simulink model "Hybrid2_modified"  (R2025a)
settings: Solver=FixedStepAuto  StartTime=0.0  StopTime=1.0  FixedStep=Ts  RelTol=1e-3
undefined symbols (not defined in the file or in its folder): closedLoop, controller, D1, D11, Delta, DiscIntNeverNeededParam, find_system, grid, level, protection, sensor, solarPanel, solarPlant, Ts
libraries: powerlib_extras x38, nesl_utility x29, spsSampleandHoldLib x24, spsThyristorLib x24, spsSeriesRLCBranchLib x23, simulink x22, fl_lib x18, ee_lib x12, spsEdgeDetectorLib x12, spsParallelRLCBranchLib x10, spsThreePhaseVIMeasurementLib x9, simulink_extras x8
(part 1 of 8)
settings Model: Creator=ELMAN  LastModifiedBy=FX
settings OptimizationCC: SimCompilerOptimization=on

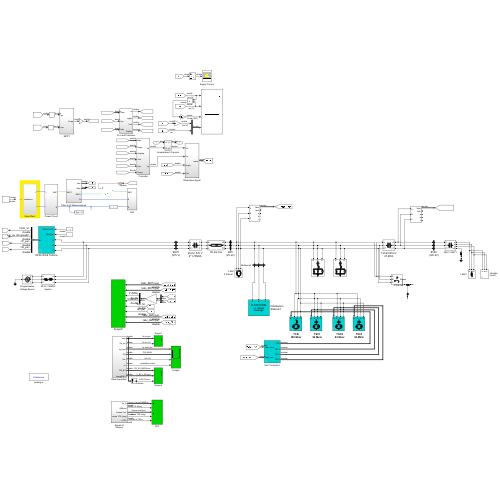
[thumbnail: Simulink's stored preview of the top-level diagram]
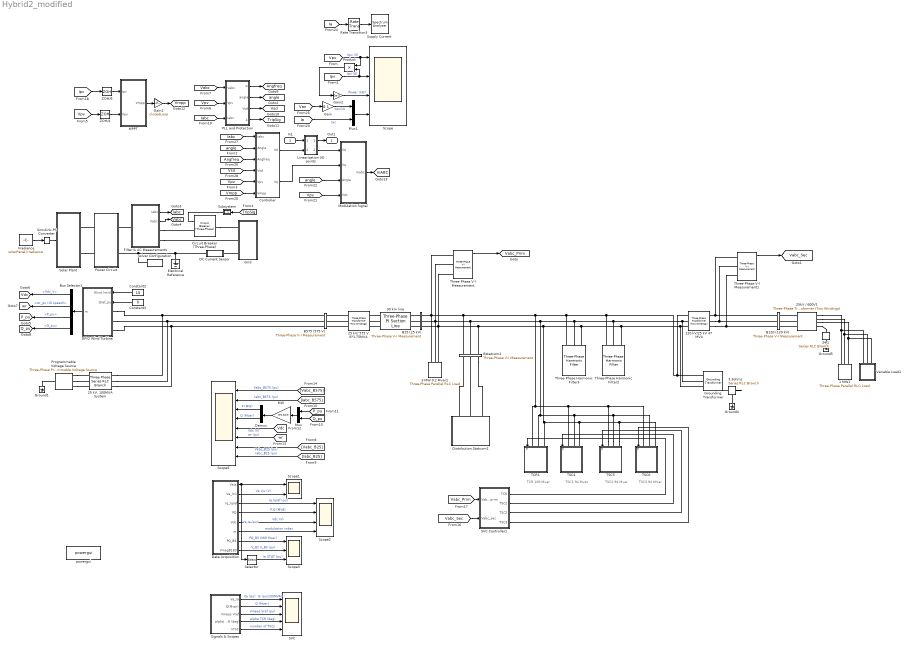
== system Hybrid2_modified ==
  note: TCR
      | 109 Mvar
  note: TSC1
      | 94 Mvar
  note: TSC2
      | 94 Mvar
  note: TSC3
      | 94 MVar
  In1 : Inport
  1 MW1 : spsThreePhaseParallelRLCLoadLib/Three-Phase Parallel RLC Load  LConnTagsString=A|B|C  Configuration=Y (floating)  NominalVoltage=600  Vabc=[1e3 1e3 1e3]  Vabcp=[1e3 1e3 1e3]  NominalFrequency=60  UnbalancedPower=off  ActivePower=1e6  InductivePower=0  CapacitivePower=0  Pabc=[10e3 9e3 11e3]  QLabc=[100 90 110]  QCabc=[100 90 110]  Pabcp=[10e3 9e3 11e3]  QLabcp=[100 90 110]  QCabcp=[100 90 110]  Measurements=None  LoadType=constant Z
  120 kV/25 kV 47 MVA : spsThreePhaseTransformerTwoWindingsLib/Three-Phase Transformer (Two Windings)  Winding1Connection=Yg  Winding2Connection=Delta (D1)  CoreType=Three single-phase transformers  SetSaturation=off  Hysteresis=off  DataFile='basic_model'  SetInitialFlux=off  Measurements=None  UNITS=pu  NominalPower=[47e6 60 ]  Winding1="[ 120e3  0.08/30   0.08 ]"  Winding2="[ 25e3  0.08/30  0.08]"  Rm=500  Lm=500  L0=0.5  Saturation="[ 0,0  ;  0.005,1.2  ;  1.0,1.4 ]"  InitialFluxes=[ 0.8 , -0.8 , 0.7 ]  BreakLoop=off  DiscreteSolver=Trapezoidal iterative  DataType=off  TransfoNumber=0
  "25 kV, 100MVA System" : spsThreePhaseSeriesRLCBranchLib/Three-Phase Series RLC Branch  LConnTagsString=A|B|C  RConnTagsString=A|B|C  BranchType=RL  Resistance=25e3^2/100e6/10  Inductance=25e3^2/100e6/(2*pi*60)  Capacitance=1.0  Measurements=None
  25 kV/ 575 V 6*1.75MVA : spsThreePhaseTransformerTwoWindingsLib/Three-Phase Transformer (Two Windings)  Winding1Connection=Delta (D11)  Winding2Connection=Yg  CoreType=Three single-phase transformers  SetSaturation=off  Hysteresis=off  DataFile='hysteresis'  SetInitialFlux=off  Measurements=None  UNITS=pu  NominalPower="[1.75e6*6  60]"  Winding1=[25e3 , 0.025/30 , 0.025]  Winding2=[ 575, 0.025/30 , 0.025]  Rm=500  Lm=inf  L0=0.5  Saturation=[ 0,0 ; 0.0024,1.2 ; 1.0,1.52 ]  InitialFluxes=[ 0.8 , -0.8 , 0.7 ]  BreakLoop=off  DiscreteSolver=Trapezoidal iterative  DataType=off  TransfoNumber=0
  25kV / 600V1 : spsThreePhaseTransformerTwoWindingsLib/Three-Phase Transformer (Two Windings)  Winding1Connection=Delta (D11)  Winding2Connection=Yn  CoreType=Three single-phase transformers  SetSaturation=off  Hysteresis=off  DataFile='basic_model'  SetInitialFlux=off  Measurements=None  UNITS=pu  NominalPower=[6e6 60]  Winding1=[25e3 , 0.05/30/2 , 0.05]  Winding2=[600 , 0.05/30/2 , 0]  Rm=500  Lm=500  L0=0.5  Saturation="[ 0,0  ;  0.005,1.2  ;  1.0,1.4 ]"  InitialFluxes=[ 0.8 , -0.8 , 0.7 ]  BreakLoop=off  DiscreteSolver=Trapezoidal iterative  DataType=off  TransfoNumber=1
  3 MW 0.2 Mvar1 : spsThreePhaseParallelRLCLoadLib/Three-Phase Parallel RLC Load  LConnTagsString=A|B|C  Configuration=Y (grounded)  NominalVoltage=25e3  Vabc=[1e3 1e3 1e3]  Vabcp=[1e3 1e3 1e3]  NominalFrequency=60  UnbalancedPower=off  ActivePower=3e6  InductivePower=0  CapacitivePower=0.2e6  Pabc=[10e3 9e3 11e3]  QLabc=[100 90 110]  QCabc=[100 90 110]  Pabcp=[10e3 9e3 11e3]  QLabcp=[100 90 110]  QCabcp=[100 90 110]  Measurements=None  LoadType=constant Z
  "3.3ohms " : spsSeriesRLCBranchLib/Series RLC Branch  LConnTagsString=__new0  RConnTagsString=__new0  BranchType=R  Resistance=3.3  Inductance=[]  SetiL0=off  InitialCurrent=0  Capacitance=[]  Setx0=off  InitialVoltage=0  Measurements=None
  30 km line : spsThreePhasePISectionLineLib/Three-Phase PI Section Line  LConnTagsString=a|b|c  RConnTagsString=A|B|C  Length=30  Frequency=60  Resistances=[0.1153 0.413]  Inductances=[1.05e-3 3.32e-3]  Capacitances=[11.33e-009 5.01e-009]
  34.1 : spsSeriesRLCBranchLib/Series RLC Branch  LConnTagsString=__new0  RConnTagsString=__new0  BranchType=R  Resistance=34.7  Inductance=1.0  SetiL0=off  InitialCurrent=0  Capacitance=1.0  Setx0=off  InitialVoltage=0  Measurements=None
  B120 (120 kV) : spsThreePhaseVIMeasurementLib/Three-Phase V-I Measurement  VoltageMeasurement=no  SetLabelV=off  LabelV=Vabc_B120  Vpu=off  VpuLL=off  CurrentMeasurement=no  SetLabelI=on  LabelI=Iabc_B120  Ipu=off  Pbase=100e6  Vbase=120e3  OutputType=Complex  PhasorSimulation=off  PSBequivalent=0
  B25 (25 kV) : spsThreePhaseVIMeasurementLib/Three-Phase V-I Measurement  VoltageMeasurement=phase-to-ground  SetLabelV=on  LabelV=Vabc_B25  Vpu=on  VpuLL=off  CurrentMeasurement=yes  SetLabelI=on  LabelI=Iabc_B25  Ipu=on  Pbase=10e6  Vbase=25e3  OutputType=Complex  PhasorSimulation=off  PSBequivalent=0
  B575 (575 V) : spsThreePhaseVIMeasurementLib/Three-Phase V-I Measurement  VoltageMeasurement=phase-to-ground  SetLabelV=on  LabelV=Vabc_B575  Vpu=on  VpuLL=off  CurrentMeasurement=yes  SetLabelI=on  LabelI=Iabc_B575  Ipu=on  Pbase=6*1.5e6/0.9  Vbase=575  OutputType=Complex  PhasorSimulation=off  PSBequivalent=0
  Bstatcom2 : spsThreePhaseVIMeasurementLib/Three-Phase V-I Measurement  VoltageMeasurement=phase-to-ground  SetLabelV=on  LabelV=Vabc_Bstatcom  Vpu=on  VpuLL=off  CurrentMeasurement=yes  SetLabelI=on  LabelI=Iabc_Bstatcom  Ipu=on  Pbase=3e6  Vbase=25e3  OutputType=Magnitude  PhasorSimulation=off  PSBequivalent=0
  Bus Selector1 : BusSelector  OutputSignals=Vdc_V,wr_pu (IG speed),PQ_pu.P_pu,PQ_pu.Q_pu
  Circuit Breaker (Three-Phase) : ee_lib/Switches & Breakers/Circuit Breaker (Three-Phase)  R_closed=0.0001 Ohm  G_open=1e-6 1/Ohm  threshold=0.5 V  breaker_behavior=ee.enum.switches.breakerBehavior.zeroCrossingEnable
      settings: InternalSimscapePortConfiguration="{\"Bottom\":[],\"Left\":[{\"id\":\"vT\",\"label\":\"vT\",\"type\":\"input\"},{\"id\":\"N1\",\"label\":\"~1\",\"type\":\"foundation.electrical.three_phase\"}],\"Right\":[{\"id\":\"N2\",\"label\":\"~2\",\"type\":\"foundation.electrical.three_phase\"}],\"Top\":[]}"
  Constant2 : Constant  Value=15
  Constant3 : Constant  Value=0
  Controller : Subsystem
  DC Current Sensor : Subsystem
      mask Display: disp('i')
  DFIG Wind Turbine : Subsystem  LoadFcn=%find_system(gcs,'FollowLinks', 'on', 'LookUnderMasks', 'all');  mask(DFIG Wind Turbine){Nb_wt=6, ShowParameters=Generator data for 1 wind turbine, nom=[1.5e6/.9 575 1975 60], sta=[ 0.023 0.18], rot=[ 0.016 0.16], Lm=2.9, mec=[0.685 0.01 3], init=[ -0.2,0   0,0,0   0,0,0 ], Imax_grid_conv=0.8, RL_grid=[ 0.3 0.003], Vdc_nom=1150, C_DClink1=10000e-6, C_var_filter1=120e3, Pmec1=1.5e6, wind_speed_CpMax=11, wind0=11, DisplayTurbChar=off, H_WT=4.32, Ksh=1.11, D_mutual=1.5, w_wt0=1.2, torque0=0.83, Kdc=[8   400], Kgrid_side_cur_reg=[0.83 5], Kspeed=[3 0.6], Krotor_side_cur_reg=[0.6 8], Ki_QV=[0.05 20], Kp_pitch=[150], Kcompensation=[3 30], PWM_freq_grid=2700, PWM_freq_rotor=1620, pitch_max=27, pitch_rate=10}
      mask prompts: Nb_wt "Number of wind turbines:"; ShowParameters "Display:"; nom "Nom. power, L-L volt. and freq. [Pn (VA), Vs_nom (Vrms), Vr_nom (Vrms), fn (Hz)]:"; sta "Stator [ Rs,Lls ] (p.u.):"; rot "Rotor [ Rr',Llr' ] (p.u.):"; Lm "Magnetizing inductance Lm (p.u.):"; mec "Inertia constant, friction factor, and pairs of poles [ H(s)  F(p.u.)  p ]:"; init "Initial conditions [s  th  ias  ibs  ics  phaseas phasebs phasecs]:"; Imax_grid_conv "Grid-side converter maximum current (pu of generator nominal current):"; RL_grid "Grid-side coupling inductor [ L, R] (p.u.):"; Vdc_nom "Nominal DC bus voltage (V):"; C_DClink1 "DC bus capacitor (F):"; C_var_filter1 "Line filter capacitor (Q=50) (var):"; Pmec1 "Nominal mechanical output power (W):"; wind_speed_CpMax "Wind speed at nominal speed and at Cp max (must be between 6 m/s and 30 m/s) (m/s):"; wind0 "Initial wind speed (m/s):"; DisplayTurbChar "Display wind turbine power characteristics:"; H_WT "Wind turbine inertia constant H (s):"; Ksh "Shaft spring constant refer to high-speed shaft (pu of nominal mechanical torque/rad):"; D_mutual "Shaft mutual damping (pu of nominal mechanical torque/pu dw):"; w_wt0 "Turbine initial speed (pu of nominal speed):"; torque0 "Initial output torque (pu of nominal mechanical torque):"; Kdc "DC bus voltage regulator gains [Kp Ki]:"; Kgrid_side_cur_reg "Grid-side converter current regulator gains [Kp Ki]:"; Kspeed "Speed regulator gains [Kp Ki]:"; Krotor_side_cur_reg "Rotor-side converter current regulator gains [Kp Ki]:"; Ki_QV "Q and V regulator gains [Ki_var Ki_volt]:"; Kp_pitch "Pitch controller gain [Kp]:"; Kcompensation "Pitch compensation gains [Kp Ki]:"; PWM_freq_grid "Frequency of the grid-side PWM carrier (Hz):"; PWM_freq_rotor "Frequency of the rotor-side PWM carrier (Hz):"; pitch_max "Maximum pitch angle (deg):"; pitch_rate "Maximum rate of change of pitch angle (deg/s):"
      mask help: This block implements a model of a variable speed pitch controlled wind turbine using a doubly-fed induction generator (DFIG).
      mask init:
      | %Generator data
      | Pnom=nom(1)*Nb_wt;
      | Vnom=nom(2);
      | Vnom_r=nom(3);
      | Fnom=nom(4);
      | Rs=sta(1);
      | Lls=sta(2);
      | Rr=rot(1);
      | Llr=rot(2);
      | H=mec(1);
      | F=mec(2);
      | p=mec(3);
      | 
      | % Converters data
      | L_RL=RL_grid(1);
      | R_RL=RL_grid(2);
      | Q_filter=50;
      | C_DClink=C_DClink1*Nb_wt;
      | C_var_filter=C_var_filter1*Nb_wt;
      | 
      | % Controller data
      | Freq_filter=1000*10;   %Hz
      | Zeta_filter=0.707;
      | Mod_index_max_grid=1.1;   %Maximum value of modulation index for grid-side converter
      | Mod_index_max_rotor=2;   %Maximum value of modulation index for rotor-side converter
      | Lim_grid_side_cur_reg=1.1; %Limit for grid-side PI current regulator (pu)
      | Lim_rotor_side_cur_reg=0.1; %Limit for rotor-side PI current regulator (pu)
      | Min_var_reg=0.9; %Minimum output value for integral var regulator (pu)
      | Max_var_reg=1.1; %Maximum output value for integral var regulator (pu)
      | Max_speed_reg=1; %Maximum output value for PI speed regulator (pu)
      | Kp_dc=Kdc(1);
      | Ki_dc=Kdc(2);
      | Kp_grid_side_cur_reg=Kgrid_side_cur_reg(1);
      | Ki_grid_side_cur_reg=Kgrid_side_cur_reg(2);
      | Kp_speed=Kspeed(1);
      | Ki_speed=Kspeed(2);
      | Kp_compensation=Kcompensation(1);
      | Ki_compensation=Kcompensation(2);
      | Kp_rotor_side_cur_reg=Krotor_side_cur_reg(1);
      | Ki_rotor_side_cur_reg=Krotor_side_cur_reg(2);
      | Ki_var=Ki_QV(1);
      | Ki_volt=Ki_QV(2);
      | Iq_ref_limit_time_constant=0.3; %(s)
      | T_speed=5;      %s
      | Min_mag_flux=0.5;   %(pu)
      | Max_Idr_ref=0.9;    %(pu)
      | Speed_max=1.2;  %(pu)
      | Speed_min=0.7;  %(pu)
      | Pitch_time_constant=0.01;    %(s)
      | 
      | 
      | % Turbine data
      | Pmec=Pmec1*Nb_wt;
      | c1 = 0.6450;
      | c2 = 116;
      | c3 = .4;
      | c4 = 5;
      | c5 = 21;
      | c6 = .00912;  % Set Pmin in stall condition (does not vary with wind_speed_Pmax)
      | c7 = .08;
      | c8 = .035;
      | theta=0;
      | CpMax=.5;
      | lambda_CpMax=9.9495;
      | 
      | c1_c8=[c1 c2 c3 c4 c5 c6 c7 c8];
      |   
      | 
      | %   Cp = c1*(c6*lambda + (-c4 - c3*(2.5 + theta) + c2*(1/(lambda + ...
      | %   c7*(2.5 + theta)) - c8/(1 + (2.5 + theta)^3)))/exp(c5*(1/(lambda + ...
      | %   c7*(2.5 + theta)) - c8/(1 + (2.5 + theta)^3))))
      | 
      | 
      |         %%%%%%%%%%%%%%%%%%%%%%%%%%%%%%%%%%%%%%%%%%%%%%%%%%%%%%%%%%%%%%%%%%%%%%%%%%%
      |         % Operation at Cp max
      |         %%%%%%%%%%%%%%%%%%%%%%%%%%%%%%%%%%%%%%%%%%%%%%%%%%%%%%%%%%%%%%%%%%%%%%%%%%%
      |         
      |         rated_omegar=1.2;
      |         omegar = rated_omegar;
      |         
      |         % Enforce boundaries on wind speed
      |         % A warning could be displayed
      |         if wind_speed_CpMax < 6
      |             wind_speed_CpMax=6;
      |             disp('Warning: Wind speed at nominal speed and at Cp max has been set to 6 m/s')
      |         end
      |         if wind_speed_CpMax > 30
      |             wind_speed_CpMax=30;
      |             disp('Warning: Wind speed at nominal speed and at Cp max has been set to 30 m/s')
      |         end
      | 
      |         K1=lambda_CpMax/omegar*wind_speed_CpMax;
      |         
      |         % Calculation of K2 needed to get P equal to the requested value at
      |         % Cp max for the requested wind speed
      |         
      |         Prated=Pmec1*Nb_wt;
      |         P_rated_omegar_theta_zero=0.75;
      |         
      |         K2 = P_rated_omegar_theta_zero*Prated/(wind_speed_CpMax^3*CpMax);
      |         
      |         K1_K2=[K1 K2];
      |         
      |         %%%%%%%%%%%%%%%%%%%%%%%%%%%%%%%%%%%%%%%%%%%%%%%%%%%%%%%%%%%%%%%%%%%%%%%%%%%
      |         % End of calculation for operation at Cp max
      |         %%%%%%%%%%%%%%%%%%%%%%%%%%%%%%%%%%%%%%%%%%%%%%%%%%%%%%%%%%%%%%%%%%%%%%%%%%%
      |         
      | 
      | %%%%%%%%%%%%%%%%%%%%%%%%%%%%%%%%%%%%%%%%%%%%%%%%%%%%%%%%%%%%%%%%%%%%%%%%%%%
      | % Plot turbine characteristics
      | %%%%%%%%%%%%%%%%%%%%%%%%%%%%%%%%%%%%%%%%%%%%%%%%%%%%%%%%%%%%%%%%%%%%%%%%%%% 
      | 
      | DisplayTurbChar=get_param(gcb,'DisplayTurbChar');
      | if strcmp(DisplayTurbChar,'on')
      |     vect_theta = 0:2:30;
      |     
      |     vect_lambda = 1:0.2:30;
      |     
      |     clear Cp;
      |     
      |     for i=1:length(vect_theta)
      |      for j=1:length(vect_lambda)
      |                 Cp(i,j) = c1*(c6*vect_lambda(j) + (-c4 - c3*(2.5 + vect_theta(i)) + c2*(1/(vect_lambda(j) + ...
      |                 c7*(2.5 + vect_theta(i))) - c8/(1 + (2.5 + vect_theta(i))^3)))/exp(c5*(1/(vect_lambda(j) + ...
      |                 c7*(2.5 + vect_theta(i))) - c8/(1 + (2.5 + vect_theta(i))^3))));
      |      end
      |     end
      | 
      |     figure(1);
      |     clf;
      |     hold on;
      | 
      |     plot(vect_lambda, Cp);
      |     axis([0, 25, 0, .6]);
      |     title('Wind Turbine Cp Characteristic (pitch angle increases by step of 2 deg.)');
      |     ylabel('Cp');
      |     set(gca,'ytick',[0 .1 .2 .3 .4 .5 .6]);
      |     xlabel('Lambda');
      |     grid on;
      |     text(10.1,0.51,'Pitch angle 0 degree');
      | 
      |     hold off
      |     
      |     % Plot of the wind turbine mechanical power output (pu) lambda and Cp
      |     % characteristics against wind speed (m/s) for a range of theta.
      |     
      |     wind_speed_range = [1,.2,30];
      |     vect_wind_speed = 1:0.2:30;
      |     
      |     clear lambda;
      |     clear Cp;
      |     clear P;
      | 
      |     for i=1:length(vect_theta)
      |         for j=1:length(vect_wind_speed)
      |             lambda(i,j) = K1*omegar/vect_wind_speed(j);
      |             Cp(i,j) = c1*(c6*lambda(i,j) + (-c4 - c3*(2.5 + vect_theta(i)) + c2*(1/(lambda(i,j) + ...
      |             c7*(2.5 + vect_theta(i))) - c8/(1 + (2.5 + vect_theta(i))^3)))/exp(c5*(1/(lambda(i,j) + ...
      |             c7*(2.5 + vect_theta(i))) - c8/(1 + (2.5 + vect_theta(i))^3))));
      |             P(i,j) = K2/Prated*vect_wind_speed(j)^3*Cp(i,j);
      |         end
      |     end
      |     
      |     
      |     figure(2);
      |     clf;
      |     hold on
      |     
      |     subplot(3,1,1);
      |     plot(vect_wind_speed, P);
      |     axis([0, 35, 0, 1.5]);
      |     title('Wind Turbine Characteristics (w = 1.2 pu, pitch angle increases by step of 2 deg.)');
      |     ylabel('P (pu)');
      |     set(gca,'ytick',0:.5:4);
      |     grid on;
      |     
      |     subplot(3,1,2);
      |     plot(vect_wind_speed, lambda);
      |     axis([0, 35, 0, 20]);
      |     ylabel('Lambda');
      |     grid on;
      |     
      |     subplot(3,1,3)
      |     plot(vect_wind_speed, Cp);
      |     axis([0, 35, 0, .6]);
      |     xlabel('Wind Speed (m/s)');
      |     ylabel('Cp');
      |     set(gca,'ytick',[0 .1 .2 .3 .4 .5 .6]);
      |     grid on;
      | 
      |     hold off
      |     set_param(gcb,'DisplayTurbChar','off')
      |     
      | end
      mask TypeOptions ShowParameters: Generator data for 1 wind turbine | Converters data for 1 wind turbine | Turbine data for 1 wind turbine | Drive train data for 1 wind turbine | Control parameters for 1 wind turbine
      mask Callback ShowParameters:
      | BlockName=getfullname(gcb);
      | %
      | Param_Show=get_param(BlockName,'ShowParameters');
      | Param_DisplayTurbChar=get_param(BlockName,'DisplayTurbChar');
      | 
      | p_mask{3}='off';p_mask{4}='off';p_mask{5}='off';
      | p_mask{6}='off';p_mask{7}='off';p_mask{8}='off';p_mask{9}='off';
      | p_mask{10}='off';p_mask{11}='off';p_mask{12}='off';p_mask{13}='off';
      | p_mask{14}='off';p_mask{15}='off';p_mask{16}='off';p_mask{17}='off';
      | p_mask{18}='off';p_mask{19}='off';p_mask{20}='off';p_mask{21}='off';
      | p_mask{22}='off';p_mask{23}='off';p_mask{24}='off';p_mask{25}='off';
      | p_mask{26}='off';p_mask{27}='off';p_mask{28}='off';p_mask{29}='off';
      | p_mask{30}='off';p_mask{31}='off';p_mask{32}='off';p_mask{33}='off';
      | 
      | 
      | switch Param_Show
      | 	case 'Generator data for 1 wind turbine'
      | 		p_mask{3}='on';p_mask{4}='on';p_mask{5}='on'; p_mask{6}='on';
      |         p_mask{7}='on'; p_mask{8}='on';
      |     case 'Converters data for 1 wind turbine'
      | 		p_mask{9}='on';p_mask{10}='on';p_mask{11}='on';p_mask{12}='on';
      |         p_mask{13}='on';
      | 	case 'Turbine data for 1 wind turbine'
      |         p_mask{14}='on';p_mask{15}='on';p_mask{16}='on';p_mask{17}='on';
      |     case 'Drive train data for 1 wind turbine'
      |         p_mask{18}='on';p_mask{19}='on';p_mask{20}='on';p_mask{21}='on';
      |         p_mask{22}='on';
      |     case 'Control parameters for 1 wind turbine'
      |         p_mask{23}='on';p_mask{24}='on';p_mask{25}='on';
      |         p_mask{26}='on';p_mask{27}='on';p_mask{28}='on';p_mask{29}='on';
      |         p_mask{30}='on'; p_mask{31}='on';p_mask{32}='on'; p_mask{33}='on';
      | end
      | 
      | ParVisible={'on','on',p_mask{3},p_mask{4},p_mask{5},p_mask{6},p_mask{7},...
      |     p_mask{8},p_mask{9},p_mask{10},p_mask{11},p_mask{12},p_mask{13},...
      |     p_mask{14},p_mask{15},p_mask{16},p_mask{17},p_mask{18},p_mask{19},...
      |     p_mask{20},p_mask{21},p_mask{22},p_mask{23},p_mask{24},p_mask{25},...
      |     p_mask{26},p_mask{27},p_mask{28},p_mask{29},p_mask{30},p_mask{31},...
      |     p_mask{32},p_mask{33}};
      | %
      | set_param(BlockName,'MaskVisibilities',ParVisible);
      | set_param(BlockName,'DisplayTurbChar',Param_DisplayTurbChar);
  Data Acquisition : Subsystem
  Demux : Demux  Outputs=2
  Distribution Statcom1 : Subsystem
      mask Display: disp('D-STATCOM\n+/- 3Mvar\nAverage')
  Electrical Reference : fl_lib/Electrical/Electrical Elements/Electrical Reference
  Filter & AC Measurements : Subsystem
  Gain : Gain  Gain=0.1
  Gain1 : Gain  Gain=closedLoop
  Gain2 : Gain  Gain=1e-3
  Grid : Subsystem
  Ground1 : spsGroundLib/Ground  LConnTagsString=a
  Ground4 : spsGroundLib/Ground  LConnTagsString=a
  Ground5 : spsGroundLib/Ground  LConnTagsString=a
  "Grounding Transformer " : spsGroundingTransformerLib/Grounding Transformer   UNITS=pu  NominalPower="[100e6   60]"  NominalVoltage=25e3  ZeroSequenceImpedance_pu=[0.025 0.75]  MagnetizationBranch_pu=[500 500]  ZeroSequenceImpedance_SI=[0.052083 589.05]  MagnetizationBranch_SI=[1041.7 3.927e+005]  Measurements=None
  Irradiance : Constant  Value=solarPanel.irradiance
  Linearization I/O points : Subsystem
  MPPT : Subsystem
  MW : Gain  Gain=6*1.5/0.9  SaturateOnIntegerOverflow=on  OutDataTypeStr=Inherit: Same as input  ParamDataTypeStr=Inherit: Same as input
  Modulation Signal : Subsystem
  Mux : Mux  Inputs=2
  Mux1 : Mux  Inputs=2
  PLL and Protection : Subsystem
  Power Circuit : Subsystem
  Product : Product
  Programmable Voltage Source : spsThreePhaseProgrammableVoltageSourceLib/Three-Phase Programmable Voltage Source  PositiveSequence=[1.077*25e3 19 60]  VariationEntity=Amplitude  VariationType=Table of time-amplitude pairs  VariationTypeAlt=Step  VariationStep=0.5  VariationRate=10  VariationMagnitude=0.3  VariationFrequency=2  VariationTiming=[1 2]  VariationPhaseA=off  Amplitudes=[1 1.06 0.94 1.0]  TimeValues="[0 0.2  0.3   0.4 ]"  HarmonicGeneration=off  HarmonicA=[3 0.2 -25 0]  HarmonicB=[2 0.15 35 2]  Timing="[0.05  3]"  BusType=swing  Pref=0  Qref=0  Qmin=-inf  Qmax=inf
  Rate Transition3 : RateTransition  OutPortSampleTime=1/(5*solarPlant.switchFrequency)
  SVC : Scope  NumInputPorts=5
      settings: SampleTime=Ts  TimeSpan=0.5993512312472854  ActiveDisplayYMinimum=-4  ActiveDisplayYMaximum=4  DataLoggingVariableName=VIabc_Prim
  SVC Controller1 : Subsystem  mask(SVC Controller){OpMode=Voltage regulation, Vref=1.0, KpKi=[0 800], Xs=0.01, Bmin_max=[-1.04  3.23], Bref=0, Ts=Ts}
      mask prompts: OpMode "Operation mode"; Vref "Reference voltage (pu):"; KpKi "Regulator gains [ Kp  Ki ]:"; Xs "Droop (pu/100MVA):"; Bmin_max "Min. and max. primary susceptances [ Bind Bcap] (pu/100MVA):"; Bref "Susceptance Bref (pu/100MVA) (Var control mode):"; Ts "Sample time (s):"
      mask help:
      | This block implements a controller for a Static Var Compensator (SVC) consisting of one thyristor-controlled reactor bank (TCR) and three thyristor-switched capacitor banks (TSCs). Outputs TCR, TSC1, TSC2 and TSC3 are vectors of six pulses for the TCR and the three TSCs.
      | In Voltage control mode the primary voltage (Vabc_prim) is controlled at Vref within the maximum inductive and capacitive susceptance range and droop setting. In Var control mode the SVC susceptance  is  kept constant at Bref (Bref<0 for inductive mode).
      | Thyristor pulses are synchronized on secondary line-to-line voltages (Vabc_sec) of the coupling transformer, assuming a Wye/Delta (D1) connection.
      mask init:
      | Kp=KpKi(1);
      | Ki=KpKi(2);
      | Bmin=Bmin_max(1);
      | Bmax=Bmin_max(2);
      mask TypeOptions OpMode: Voltage regulation | Var control (Fixed susceptance Bref)
  Scope : Scope  NumInputPorts=4
      settings: TimeSpan=simulation.timeSim  ActiveDisplayYMinimum=-178.21524004215382  ActiveDisplayYMaximum=1603.9371603793847
  Scope1 : Scope  NumInputPorts=2
      settings: SampleTime=Ts  TimeSpan=0.5  ActiveDisplayYMinimum=-1.5  ActiveDisplayYMaximum=1.5  DataLoggingVariableName=Sig1
  Scope2 : Scope  NumInputPorts=4
      settings: SampleTime=Ts*32  TimeSpan=0.5  ActiveDisplayYMinimum=-2.0010436377768239  ActiveDisplayYMaximum=1.7915582294498202  DataLoggingVariableName=Sig2
  Scope3 : Scope  NumInputPorts=3
      settings: SampleTime=Ts  TimeSpan=0.5  ActiveDisplayYMinimum=-1  ActiveDisplayYMaximum=1  DataLoggingVariableName=Sig
  Scope5 : Scope  NumInputPorts=8
      settings: TimeSpan=0.2  ActiveDisplayYMinimum=-2  ActiveDisplayYMaximum=2  DataLoggingVariableName=ScopeData2  DataLoggingSaveFormat=Array
  Selector : Selector  InputPortWidth=2  IndexOptions=Index vector (dialog)  Indices=2  OutputSizes=1
  Signals & Scopes : Subsystem
  Simulink-PS Converter : nesl_utility/Simulink-PS Converter  PhysicalDomain=network_engine_domain  SubClassName=ps_input  LeftPortType=input  RightPortType=output  PseudoPeriodic=off  Frequencies=[]  NoiseDistribution=none  NoiseParameters=[]  Unit=1  AffineConversion=off  FilteringAndDerivatives=provide  SimscapeFilterOrder=1  InputFilterTimeConstant=0.001  UdotUserProvided=0
  Solar Plant : Subsystem
  Solver Configuration : nesl_utility/Solver Configuration  PhysicalDomain=network_engine_domain  SubClassName=solver  LeftPortType=input  RightPortType=generic  Tones=[]  Harmonics=[]  SimulateNoise=off  Profile=off  UseLocalSampling=off  EnableSwitchedLinearOptims=on  FrequencyDomain=off  UseCCode=off  RelTol=0.001  AbsTol=1e-06  MinStep=1e-09  ToWorkspace=off  RevertToSquareIcSolve=off  NumHomotopyIterations=100  PhasorMode=off  PhasorModeNumHarmonics=1  ConsistencySolver=NEWTON_FTOL  IndexReductionMethod=DerivativeReplacement  DoDC=off  ResidualTolerance=1e-9  ConsistencyTolSource=GLOBAL  ConsistencyAbsTol=0.001  ConsistencyRelTol=0.001  ConsistencyTolFactor=0.001  UseLocalSolver=off  LocalSolverChoice=NE_TRAPEZOIDAL_ADVANCER  ResolveIndetEquations=on  FunctionEvalNumThread=1  LocalSolverSampleTime=1e-7  DoFixedCost=off  MaxNonlinIter=10  MaxModeIter=2  ComputeImpulses=off  ImpulseIterations=2  LinearAlgebra=auto  LinearAlgebraNumThread=0  EquationFormulation=NE_TIME_EF  DelaysMemoryBudget=1024  AutomaticFiltering=on  FilteringTimeConstant=0.001  PartitionStorageMethod=AS_NEEDED  PartitionMemoryBudget=1024  PartitionMethod=FAST  MultibodyUseLocalSolver=off  MultibodyLocalSolverChoice=ODE1  MultibodyLocalSolverSampleTime=0.001
  Subsystem : Subsystem
  Supply Current : SpectrumAnalyzer  WindowPosition=[1059 553 620 438]  ScopeFrameLocation=window  SpectrumType=RMS  Method=Welch  SampleRate=100000  PlotAsTwoSidedSpectrum=off  FrequencyScale=Log  AxesScaling=Manual  RBWSource=Property  RBW=9  Span=50000  CenterFrequency=25000  StartFrequency=0  StopFrequency=50000  OverlapPercent=90  AveragingMethod=Running  SpectrumUnits=Vrms  YLimits=[-4.5063154233397524351,40.557285835884592018]  ColorLimits=[0.0061790664803535039207,16.888204283875005274]  AllowFFTLengthLessThanSamplesPerUpdate=on
      settings: OpenAtSimulationStart=off
  TCR1 : Subsystem  LoadFcn=find_system(gcs,'FollowLinks', 'on', 'LookUnderMasks', 'all');  mask(TCR branch){Ltcr=18.7e-3, Q=50, ParS=[500 250e-9], ParT=[1e-3  1*15]}
      mask prompts: Ltcr "TCR Inductance (H) :"; Q "Quality factor:"; ParS "Thyristor snubber: [ R (ohm)   C (F)  ]"; ParT "Thyristor data: [ Ron (ohm)   Vf (volt) ]"
      mask init:
      | Rtcr=(2*pi*60) * Ltcr / Q;
      | Rsnub=ParS(1);
      | Csnub=ParS(2);
      | Ron=ParT(1);
      | Vf=ParT(2);
      mask Display:
      | plot(0,0);plot(125,220)
      | plot([62 62 37 37 49 25 37],[15 39 39 58 76 76 58])
      | plot([62 87 87 99 87 75 87],[39 39 58 58 76 58 58])
      | plot([25 49],[58 58]);plot([37 25],[58 49])
      | plot([75 99],[76 76]);plot([87 99],[76 85])
      | plot([37 37 87 87],[76 95 95 76])
      | plot([62 62],[95 122]);plot([62 62],[164 186])
      | plot([62 72 78 79 78 72 62],[122 123 125 129 133 135 136])
      | plot([62 72 78 79 78 72 62],14+[122 123 125 129 133 135 136])
      | plot([62 72 78 79 78 72 62],28+[122 123 125 129 133 135 136])
  TSC4 : Subsystem  mask(TSC branch){Ccmt=308.4e-6, ParL=[1.13e-3 4.26e-3*2 191.7/2], ParS=[500 250e-9], ParT=[1e-3  1*15]}
      mask prompts: Ccmt "Capacitance (F) :"; ParL "[ Inductance (H)  Rseries (ohm)  Rparallel (ohm)  ]"; ParS "Thyristor snubber: [ R (ohm)   C (F)  ]"; ParT "Thyristor data: [ Ron (ohm)  Vf (volt) ]"
      mask init:
      | Lcmt=ParL(1);
      | Rseries=ParL(2);
      | Rparallel=ParL(3);
      | Rsnub=ParS(1);
      | Csnub=ParS(2);
      | Ron=ParT(1);
      | Vf=ParT(2);
      mask Display:
      | plot(0,0);plot(125,220)
      | plot([62 62 37 37 49 25 37],[15 39 39 58 76 76 58])
      | plot([62 87 87 99 87 75 87],[39 39 58 58 76 58 58])
      | plot([25 49],[58 58]);plot([37 25],[58 49])
      | plot([75 99],[76 76]);plot([87 99],[76 85])
      | plot([37 37 87 87],[76 95 95 76])
      | plot([62 62],[95 133]);plot([62 62],[164 183])
      | plot([62 69 73 78 81 82],13+[120 120 119 118 117 115])
      | plot([62 55 51 46 43 42],13+[120 120 119 118 117 115])
      | plot([42 82],[145 145])
      | plot([62 62],[145 164])
  TSC5 : Subsystem  mask(TSC branch){Ccmt=308.4e-6, ParL=[1.13e-3 4.26e-3*2 191.7/2], ParS=[500 250e-9], ParT=[1e-3 1*15]}
      mask prompts: Ccmt "Capacitance (F) :"; ParL "[ Inductance (H)  Rseries (ohm)  Rparallel (ohm)  ]"; ParS "Thyristor snubber: [ R (ohm)   C (F)  ]"; ParT "Thyristor data: [ Ron (ohm)  Vf (volt) ]"
      mask init:
      | Lcmt=ParL(1);
      | Rseries=ParL(2);
      | Rparallel=ParL(3);
      | Rsnub=ParS(1);
      | Csnub=ParS(2);
      | Ron=ParT(1);
      | Vf=ParT(2);
      mask Display:
      | plot(0,0);plot(125,220)
      | plot([62 62 37 37 49 25 37],[15 39 39 58 76 76 58])
      | plot([62 87 87 99 87 75 87],[39 39 58 58 76 58 58])
      | plot([25 49],[58 58]);plot([37 25],[58 49])
      | plot([75 99],[76 76]);plot([87 99],[76 85])
      | plot([37 37 87 87],[76 95 95 76])
      | plot([62 62],[95 133]);plot([62 62],[164 183])
      | plot([62 69 73 78 81 82],13+[120 120 119 118 117 115])
      | plot([62 55 51 46 43 42],13+[120 120 119 118 117 115])
      | plot([42 82],[145 145])
      | plot([62 62],[145 164])
  TSC6 : Subsystem  mask(TSC branch){Ccmt=308.4e-6, ParL=[1.13e-3 4.26e-3*2 191.7/2], ParS=[500 250e-9], ParT=[1e-3 1*15]}
      mask prompts: Ccmt "Capacitance (F) :"; ParL "[ Inductance (H)  Rseries (ohm)  Rparallel (ohm)  ]"; ParS "Thyristor snubber: [ R (ohm)   C (F)  ]"; ParT "Thyristor data: [ Ron (ohm)  Vf (volt) ]"
      mask init:
      | Lcmt=ParL(1);
      | Rseries=ParL(2);
      | Rparallel=ParL(3);
      | Rsnub=ParS(1);
      | Csnub=ParS(2);
      | Ron=ParT(1);
      | Vf=ParT(2);
      mask Display:
      | plot(0,0);plot(125,220)
      | plot([62 62 37 37 49 25 37],[15 39 39 58 76 76 58])
      | plot([62 87 87 99 87 75 87],[39 39 58 58 76 58 58])
      | plot([25 49],[58 58]);plot([37 25],[58 49])
      | plot([75 99],[76 76]);plot([87 99],[76 85])
      | plot([37 37 87 87],[76 95 95 76])
      | plot([62 62],[95 133]);plot([62 62],[164 183])
      | plot([62 69 73 78 81 82],13+[120 120 119 118 117 115])
      | plot([62 55 51 46 43 42],13+[120 120 119 118 117 115])
      | plot([42 82],[145 145])
      | plot([62 62],[145 164])
  Three-Phase Harmonic Filter2 : spsThreePhaseHarmonicFilterLib/Three-Phase Harmonic Filter  LConnTagsString=A|B|C  RConnTagsString=n  FilterType=Double-tuned  FilterConnection=Y (neutral)  ParNom=[315e3 60]  Qc=49e6  Fr=[5*60]  Frd=[11*60 13*60]  Q=16  Measurements=None
      settings: AttributesFormatString=\n
      settings: LibrarySourceBlock=|
      | sps_lib/Passives/Three-Phase
      | Harmonic Filter
  Three-Phase Harmonic Filter3 : spsThreePhaseHarmonicFilterLib/Three-Phase Harmonic Filter  LConnTagsString=A|B|C  RConnTagsString=n  FilterType=Double-tuned  FilterConnection=Y (neutral)  ParNom=[315e3 60]  Qc=49e6  Fr=[5*60]  Frd=[11*60 13*60]  Q=16  Measurements=None
      settings: AttributesFormatString=\n
      settings: LibrarySourceBlock=|
      | sps_lib/Passives/Three-Phase
      | Harmonic Filter
  Three-Phase V-I Measurement : spsThreePhaseVIMeasurementLib/Three-Phase V-I Measurement  VoltageMeasurement=phase-to-ground  SetLabelV=off  LabelV=Vabc  Vpu=off  VpuLL=off  CurrentMeasurement=yes  SetLabelI=off  LabelI=Iabc  Ipu=off  Pbase=100e6  Vbase=500e3  OutputType=Complex  PhasorSimulation=off  PSBequivalent=0
  Three-Phase V-I Measurement1 : spsThreePhaseVIMeasurementLib/Three-Phase V-I Measurement  VoltageMeasurement=phase-to-ground  SetLabelV=off  LabelV=Vabc  Vpu=off  VpuLL=off  CurrentMeasurement=yes  SetLabelI=off  LabelI=Iabc  Ipu=off  Pbase=100e6  Vbase=500e3  OutputType=Complex  PhasorSimulation=off  PSBequivalent=0
  Variable Load1 : Subsystem  mask(Variable Load (Constant Current)){Par_Nom=[3000 0.9], Par_Mod=[2000  5], Par_Time=[0.15 1]*100, Vbase=600, Ts=Ts}
      mask prompts: Par_Nom "Nominal load: [ Current (Arms)    Power factor (0 a 1) ]"; Par_Mod "Modulation: [ Amplitude (Arms)   Frequency (Hz) ]"; Par_Time "Modulation timing : [ Ton  Toff ]"; Vbase "Nominal voltage (Volts rms ph-ph)"; Ts "Sample time:"
      mask init:
      | NomAmp=Par_Nom(1)*sqrt(2);
      | NomPha=-acos(Par_Nom(2));
      | ModFreq=Par_Mod(2);
      | ModAmp=Par_Mod(1)*sqrt(2);
      | Ton=Par_Time(1);
      | Toff=Par_Time(2);
  ZOH/4 : ZeroOrderHold  SampleTime=solarPlant.timeMPPT
  ZOH/6 : ZeroOrderHold  SampleTime=solarPlant.timeMPPT
  powergui : spspowerguiLib/powergui  Priority=2  SimulationMode=Continuous  SampleTime=Ts  frequency=60  Iterations=50  frequencyindice=0  Pbase=100e6  ErrMax=1e-4  UnitsV=kV  UnitsW=MW  buscounter=0  FunctionMessages=off  echomessages=off  EnableUseOfTLC=off  CurrentSourceSwitches=off  DisableSnubberDevices=off  DisableRonSwitches=off  DisableVfSwitches=off  DisplayEquations=off  AutomaticDiscreteSolvers=off  SolverType=Tustin/Backward Euler (TBE)  Interpol=off  ExternalGateDelay=off  methode=off  Ts=0  x0status=blocks  SPID=off  SwTol=0  HookPort=off  NonlinearTolerance=1e-4  nMaxIteration=100  ContinueOnMaxIteration=off  RestoreLinks=warning  ResistiveCurrentMeasurement=off  Frange=[0:2:500]  Ylog=off  Xlog=on  ShowGrid=off  save=off  variable=ZData  structure=Sig1  ZoomFFT=on  StartTime=0.26  cycles=2  DisplayStyle=1  fundamental=60  FreqAxis=off  MaxFrequency=5000  frequencyindicesteady=1  RmsSteady=1  display=off
  Out1 : Outport  VectorParamsAs1DForOutWhenUnconnected=off
  tag scope: Angfreq=global, Iabc=global, P_pu=global, Q_pu=global, TripSig=global, Vabc=global, Vabc_Prim=global, Vabc_Sec=global, Vdc=global, Vmpp=global, Vsd=global, angle=global, mABC=global, wr=global
  wires:
  Selector/1 -> Scope3/3  "Ia STAT (pu)"
  Data Acquisition/8(VmagB1B3) -> Scope3/2  "V_B1 V_B3 (pu)"
  Data Acquisition/6(m) -> Scope2/4  "modulation index"
  Data Acquisition/4(PQ) -> Scope2/2  "P,Q (MVA)"
  Data Acquisition/1(VaIa) -> Scope1/1, Selector/1  "Va,Ia (pu)"
  Data Acquisition/3(Iq_Iqref) -> Scope2/1  "Iq,Iqref (pu)"
  Data Acquisition/2(Va_Inv) -> Scope1/2  "Va Inv (V)"
  Data Acquisition/5(Vdc) -> Scope2/3  "Vdc (V)"
  Data Acquisition/7(PQ_B3) -> Scope3/1  "PQ_B3 (MW Mvar)"
  Signals & Scopes/3("Vmeas Vref ") -> SVC/3  "Vmeas Vref (pu)"
  Signals & Scopes/4(alpha TCR (deg)) -> SVC/4  "alpha TCR (deg)"
  Signals & Scopes/5(nTSC) -> SVC/5  "number of TSCs"
  Signals & Scopes/2(Q(Mvar)) -> SVC/2  "Q (Mvar)"
  Signals & Scopes/1(Va_Ia) -> SVC/1  "Va (pu)  Ia (pu/100MVA)"
  DFIG Wind Turbine/1(m) -> Bus Selector1/1
  [Iabc_B575] -> Scope5/2  "Iabc_B575 (pu)"
  [P_pu] -> Mux/1
  Bus Selector1/4 -> [Q_pu]  "<Q_pu>"
  Bus Selector1/3 -> [P_pu]  "<P_pu>"
  Mux/1 -> MW/1
  [wr] -> Scope5/6  "wr (pu)"
  Demux/1 -> Scope5/3  "P (MW)"
  Bus Selector1/1 -> [Vdc]  "<Vdc_V>"
  [Iabc_B25] -> Scope5/8  "Iabc_B25 (pu)"
  Bus Selector1/2 -> [wr]  "<wr_pu (IG speed)>"
  [Q_pu] -> Mux/2
  [Vdc] -> Scope5/5  "Vdc (V)"
  Demux/2 -> Scope5/4  "Q (Mvar)"
  [Vabc_B575] -> Scope5/1  "Vabc_B575 (pu)"
  Constant2/1 -> DFIG Wind Turbine/1("Wind (m/s) ")
  [Vabc_B25] -> Scope5/7  "Vabc_B25 (pu)"
  Constant3/1 -> DFIG Wind Turbine/2(Qref_pu)
  MW/1 -> Demux/1
  SVC Controller1/4(TSC3) -> TSC6/1(P)
  SVC Controller1/3(TSC2) -> TSC5/1(P)
  SVC Controller1/1(TCR) -> TCR1/1(P)
  SVC Controller1/2(TSC1) -> TSC4/1(P)
  [Vabc_Sec] -> SVC Controller1/2(Vabc_sec)
  [Vabc_Prim] -> SVC Controller1/1(Vabc_prim)
  Three-Phase V-I Measurement/1 -> [Vabc_Prim]
  Three-Phase V-I Measurement1/1 -> [Vabc_Sec]
  [Vpv] -> Controller/5(Vpv)
  [Ipv] -> ZOH/6/1
  Modulation Signal/1(mabc) -> [mABC]
  [Vsd] -> Controller/4(Vsd)
  [Angfreq] -> Controller/3(Angfreq)
  Mux1/1 -> Scope/4
  Filter & AC Measurements/1(Iabc) -> [Iabc]
  [angle] -> Controller/2(Angle)
  [Vabc] -> PLL and Protection/1(Vabc)
  [Vpv] -> ZOH/4/1
  [Van] -> Gain/1
  PLL and Protection/4(TripSig) -> [TripSig]
  Linearization I/O points/2(y1) -> Modulation Signal/1(Vd)
  Gain1/1 -> [Vmpp]
  ZOH/4/1 -> MPPT/2(Vpv)
  Linearization I/O points/1(y2) -> Out1/1
  Irradiance/1 -> Simulink-PS Converter/1
  [angle] -> Modulation Signal/3(Angle)
  [Vpv] -> Product/1, Scope/1  "Vpv (V)"
  Gain2/1 -> Scope/3  "Power (kW)"
  Controller/2(Vq) -> Modulation Signal/2(Vq)
  [Vpv] -> PLL and Protection/2(Vpv)
  MPPT/1(Vmpp) -> Gain1/1
  PLL and Protection/1(w) -> [Angfreq]
  Filter & AC Measurements/2(Vabc) -> [Vabc]
  [TripSig] -> Subsystem/1(i)
  PLL and Protection/2(angle) -> [angle]
  [Iabc] -> Controller/1(Iabc)
  [Ia] -> Mux1/2  "Iac"
  In1/1 -> Linearization I/O points/1(u2)
  Rate Transition3/1 -> Supply Current/1
  ZOH/6/1 -> MPPT/1(Ipv)
  [Vmpp] -> Controller/6(Vmpp)
  PLL and Protection/3(Vsd) -> [Vsd]
  Product/1 -> Gain2/1
  [Ipv] -> Product/2, Scope/2  "Ipv (A)"
  [Ia] -> Rate Transition3/1
  Controller/1(Vd) -> Linearization I/O points/2(u1)
  Gain/1 -> Mux1/1  "Vac/10"
  [Iabc] -> PLL and Protection/3(Iabc)
  [Vpv] -> Modulation Signal/4(Vdc)
  connections:
  Programmable Voltage Source/RConn1 -- "25 kV, 100MVA System"/LConn1
  Ground1/LConn1 -- Programmable Voltage Source/LConn1
  Programmable Voltage Source/RConn3 -- "25 kV, 100MVA System"/LConn3
  Programmable Voltage Source/RConn2 -- "25 kV, 100MVA System"/LConn2
  TSC5/LConn2 -- TSC6/LConn2 -- TSC4/LConn2 -- TCR1/LConn2 -- Three-Phase Harmonic Filter2/LConn2 -- "Grounding Transformer "/LConn2 -- 120 kV/25 kV 47 MVA/RConn2 -- Three-Phase Harmonic Filter3/LConn2 -- Bstatcom2/LConn2 -- Three-Phase V-I Measurement/LConn2 -- 3 MW 0.2 Mvar1/LConn2 -- B25 (25 kV)/LConn2
  TSC5/LConn3 -- TSC6/LConn3 -- Three-Phase Harmonic Filter2/LConn3 -- "Grounding Transformer "/LConn3 -- 120 kV/25 kV 47 MVA/RConn3 -- Three-Phase Harmonic Filter3/LConn3 -- Bstatcom2/LConn3 -- Three-Phase V-I Measurement/LConn3 -- 3 MW 0.2 Mvar1/LConn3 -- B25 (25 kV)/LConn3 -- TCR1/LConn3 -- TSC4/LConn3
  TSC5/LConn1 -- TSC4/LConn1 -- TCR1/LConn1 -- Three-Phase Harmonic Filter2/LConn1 -- "Grounding Transformer "/LConn1 -- 120 kV/25 kV 47 MVA/RConn1 -- Three-Phase Harmonic Filter3/LConn1 -- Bstatcom2/LConn1 -- B25 (25 kV)/LConn1 -- Three-Phase V-I Measurement/LConn1 -- 3 MW 0.2 Mvar1/LConn1 -- TSC6/LConn1
  25 kV/ 575 V 6*1.75MVA/RConn1 -- B575 (575 V)/LConn1
  120 kV/25 kV 47 MVA/LConn1 -- Three-Phase V-I Measurement1/LConn1 -- B120 (120 kV)/RConn1
  "3.3ohms "/RConn1 -- Ground4/LConn1
  "3.3ohms "/LConn1 -- "Grounding Transformer "/RConn1
  30 km line/RConn3 -- 25 kV/ 575 V 6*1.75MVA/LConn3
  25kV / 600V1/LConn3 -- B120 (120 kV)/LConn3
  30 km line/RConn2 -- 25 kV/ 575 V 6*1.75MVA/LConn2
  B25 (25 kV)/RConn3 -- 30 km line/LConn3
  DFIG Wind Turbine/LConn2 -- "25 kV, 100MVA System"/RConn2 -- B575 (575 V)/RConn2
  120 kV/25 kV 47 MVA/LConn3 -- Three-Phase V-I Measurement1/LConn3 -- B120 (120 kV)/RConn3
  DFIG Wind Turbine/LConn1 -- "25 kV, 100MVA System"/RConn1 -- B575 (575 V)/RConn1
  25 kV/ 575 V 6*1.75MVA/RConn3 -- B575 (575 V)/LConn3
  DFIG Wind Turbine/LConn3 -- "25 kV, 100MVA System"/RConn3 -- B575 (575 V)/RConn3
  30 km line/RConn1 -- 25 kV/ 575 V 6*1.75MVA/LConn1
  B25 (25 kV)/RConn2 -- 30 km line/LConn2
  25kV / 600V1/LConn2 -- B120 (120 kV)/LConn2
  120 kV/25 kV 47 MVA/LConn2 -- Three-Phase V-I Measurement1/LConn2 -- B120 (120 kV)/RConn2
  25 kV/ 575 V 6*1.75MVA/RConn2 -- B575 (575 V)/LConn2
  B25 (25 kV)/RConn1 -- 30 km line/LConn1
  Distribution Statcom1/RConn2 -- Bstatcom2/RConn2
  Bstatcom2/RConn3 -- Distribution Statcom1/RConn3
  Distribution Statcom1/RConn1 -- Bstatcom2/RConn1
  Variable Load1/LConn3 -- 25kV / 600V1/RConn3 -- 1 MW1/LConn3
  Variable Load1/LConn2 -- 25kV / 600V1/RConn2 -- 1 MW1/LConn2
  Variable Load1/LConn1 -- 25kV / 600V1/RConn1 -- 1 MW1/LConn1
  34.1/RConn1 -- Ground5/LConn1
  25kV / 600V1/RConn4 -- 34.1/LConn1
  25kV / 600V1/LConn1 -- B120 (120 kV)/LConn1
  Power Circuit/RConn2 -- Solver Configuration/RConn1 -- DC Current Sensor/RConn1 -- Electrical Reference/LConn1
  Filter & AC Measurements/LConn1 -- Power Circuit/RConn1
  Filter & AC Measurements/RConn2 -- Grid/LConn2
  Power Circuit/LConn1 -- Solar Plant/RConn1
  Simulink-PS Converter/RConn1 -- Solar Plant/LConn1
  Circuit Breaker (Three-Phase)/LConn1 -- Subsystem/RConn1
  Solar Plant/RConn2 -- Power Circuit/LConn2
  Filter & AC Measurements/RConn1 -- Circuit Breaker (Three-Phase)/LConn2
  Grid/LConn3 -- DC Current Sensor/LConn1
  Circuit Breaker (Three-Phase)/RConn1 -- Grid/LConn1

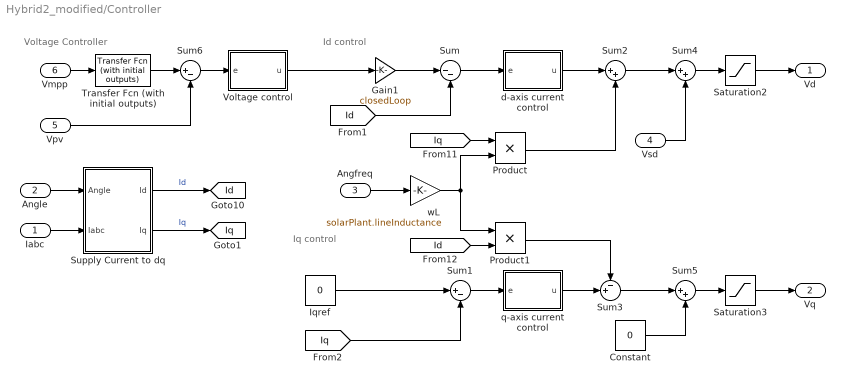
== system Hybrid2_modified/Controller ==
  note: Id control
  note: Voltage Controller
  note: Iq control
  Iabc : Inport
  Angle : Inport  Port=2
  Angfreq : Inport  Port=3
  Vsd : Inport  Port=4
  Vpv : Inport  Port=5
  Vmpp : Inport  Port=6
  Constant : Constant  Value=0
  Gain1 : Gain  Gain=closedLoop
  Iqref : Constant  Value=0
  Product : Product
  Product1 : Product
  Saturation2 : Saturate  UpperLimit=controller.currentVoltMax*1.5  LowerLimit=-1*controller.currentVoltMax*1.5
  Saturation3 : Saturate  UpperLimit=controller.currentVoltMax*1.5  LowerLimit=-1*controller.currentVoltMax*1.5
  Sum : Sum  Inputs=|--
  Sum1 : Sum  Inputs=|+-
  Sum2 : Sum  Inputs=|++
  Sum3 : Sum  Inputs=-+|
  Sum4 : Sum  Inputs=|++
  Sum5 : Sum  Inputs=|++
  Sum6 : Sum  Inputs=|+-
  Supply Current to dq : Subsystem
  Transfer Fcn (with initial outputs) : simulink_extras/Additional Linear/Transfer Fcn (with initial outputs)  N=[1]  D="[solarPlant.timeMPPT*50  1]"  Y0=solarPlant.DCMPPTValue  U0=solarPlant.DCMPPTValue
  Voltage control : Subsystem
  d-axis current control : Subsystem
  q-axis current control : Subsystem
  wL : Gain  Gain=solarPlant.lineInductance
  Vd : Outport  VectorParamsAs1DForOutWhenUnconnected=off
  Vq : Outport  Port=2  VectorParamsAs1DForOutWhenUnconnected=off
  tag scope: Id=global, Iq=global
  wires:
  Sum1/1 -> q-axis current control/1(e)
  wL/1 -> Product/2, Product1/1
  [Id] -> Product1/2
  [Iq] -> Product/1
  Product1/1 -> Sum3/1
  Product/1 -> Sum2/2
  Sum3/1 -> Sum5/1
  Sum2/1 -> Sum4/1
  Sum4/1 -> Saturation2/1
  Sum5/1 -> Saturation3/1
  Angfreq/1 -> wL/1
  Constant/1 -> Sum5/2
  Angle/1 -> Supply Current to dq/1(Angle)
  Vpv/1 -> Sum6/2
  Sum/1 -> d-axis current control/1(e)
  [Id] -> Sum/2
  d-axis current control/1(u) -> Sum2/1
  q-axis current control/1(u) -> Sum3/2
  Supply Current to dq/1(Id) -> [Id]  "Id"
  Supply Current to dq/2(Iq) -> [Iq]  "Iq"
  Iabc/1 -> Supply Current to dq/2(Iabc)
  Vsd/1 -> Sum4/2
  Sum6/1 -> Voltage control/1(e)
  Vmpp/1 -> Transfer Fcn (with initial outputs)/1
  Transfer Fcn (with initial outputs)/1 -> Sum6/1
  Saturation3/1 -> Vq/1
  Saturation2/1 -> Vd/1
  Iqref/1 -> Sum1/1
  [Iq] -> Sum1/2
  Voltage control/1(u) -> Gain1/1
  Gain1/1 -> Sum/1

== system Hybrid2_modified/DC Current Sensor ==
  note: In the transformerless grid connected PV system, leakage current depends on, PWM technique, DC bus voltage ripple, earth resistance and semi conductor switch switching time. So for accurately estimating the leakage current requires better PWM technique (bipolar PWM), DC bus voltage ripple, semi conductor model and earth resistance.
  Current Sensor : fl_lib/Electrical/Electrical Sensors/Current Sensor
      settings: LogSimulationData=on
  PS-Simulink Converter : nesl_utility/PS-Simulink Converter  PhysicalDomain=network_engine_domain  SubClassName=ps_output  LeftPortType=input  RightPortType=output  PseudoPeriodic=off  Frequencies=[]  VectorFormat=1-D array  Unit=1  AffineConversion=off
  Scope : Scope
      settings: ActiveDisplayYMinimum=-19.9023  ActiveDisplayYMaximum=7.22766  DataLoggingVariableName=ScopeData2
  Sensor dynamics : TransferFcn  Numerator=1  Denominator=[1/sensor.samplingFreq 1]
  - : PMIOPort  Side=Left
  + : PMIOPort  Port=2  Side=Right
  wires:
  PS-Simulink Converter/1 -> Sensor dynamics/1
  Sensor dynamics/1 -> Scope/1
  connections:
  Current Sensor/RConn2 -- -/RConn1
  +/RConn1 -- Current Sensor/LConn1
  Current Sensor/RConn1 -- PS-Simulink Converter/LConn1
